simulink model "generating_a_ramp"  (Simulink 6.6)
settings: Solver=VariableStepDiscrete  SolverMode=SingleTasking  StartTime=0.0  StopTime=2048/100e3  RelTol=1e-3
libraries: xbsIndex_r4 x5
settings Model: Creator=lcrockett  LastModifiedBy=lcrockett
settings DataIOCC: SignalLoggingName=sigsOut
settings OptimizationCC: InlineParams=on  InlineInvariantSignals=on
settings DebuggingCC: SignalResolutionControl=TryResolveAllWithWarning  SolverPrmCheckMsg=none  MultiTaskDSMMsg=warning  MultiTaskCondExecSysMsg=none  StrictBusMsg=None
settings HardwareCC: TargetUnknown=on
settings RTWCC: IncludeERTFirstTime=on
settings GRTTargetCC: ModelReferenceCompliant=off  MatFileLogging=off

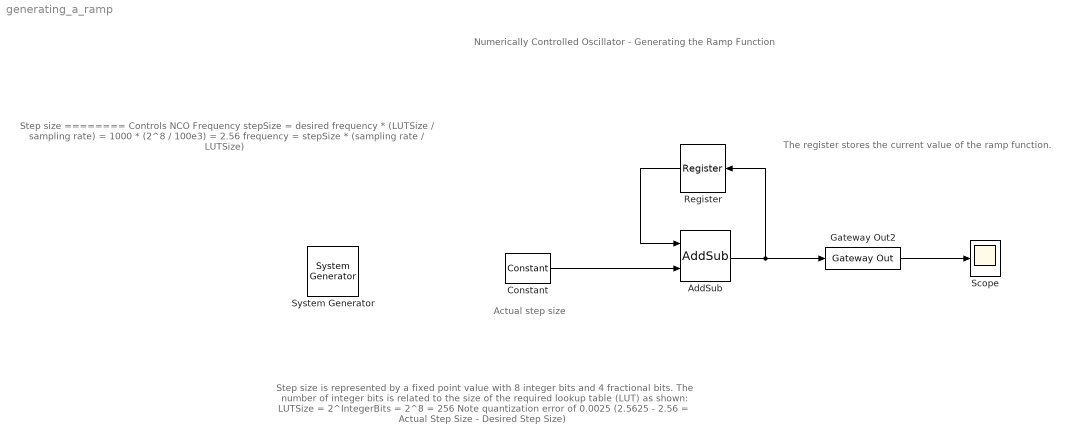
== system generating_a_ramp ==
  note: Step size
      | ========
      | Controls NCO Frequency
      |
      | stepSize =  desired frequency * (LUTSize  / sampling rate)
      |               =  1000 * (2^8  / 100e3)
      |               =  2.56
      |
      | frequency = stepSize * (sampling rate / LUTSize)
  note: The register stores the current value of the ramp function.
  note: Numerically Controlled Oscillator - Generating the Ramp Function
  note: Actual step size
  note: Step size is represented by a fixed point value with 8 integer bits and 4 fractional bits.
      | The number of integer bits is related to the size of the required lookup table (LUT) as shown:
      |
      | LUTSize = 2^IntegerBits = 2^8 = 256
      |
      | Note quantization error of 0.0025 (2.5625 - 2.56 = Actual Step Size - Desired Step Size)
  " System Generator" : xbsIndex_r4/ System Generator  Tag=genX  SystemSampleTime=-1  xilinxfamily=virtex2p  part=xc2vp30  speed=-7  package=ff896  synthesis_tool=XST  directory=./netlist  testbench=off  simulink_period=1/100e3  sysclk_period=50  incr_netlist=off  trim_vbits=Everywhere in SubSystem  dbl_ovrd=According to Block Masks  core_generation=According to Block Masks  run_coregen=off  deprecated_control=off  eval_field=0  block_type=sysgen
      settings: block_version=9.2.01
  AddSub : xbsIndex_r4/AddSub  mode=Addition  use_carryin=off  use_carryout=off  en=off  latency=0  precision=User Defined  arith_type="Signed  (2's comp)"  n_bits=12  bin_pt=4  quantization=Truncate  overflow=Wrap  dbl_ovrd=off  use_behavioral_HDL=on  pipelined=off  use_rpm=on  block_type=addsub
      settings: xl_area=[0, 0, 0, 0, 0, 0, 0]  block_version=VER_STRING_GOES_HERE
  Constant : xbsIndex_r4/Constant  arith_type=Signed (2's comp)  const=2.56  n_bits=12  bin_pt=4  explicit_period=on  period=1/100e3  equ=P=C  opselect=C  inp2=PCIN>>17  opr=+  inp1=P  carry=CIN  dbl_ovrd=off  block_type=constant
      settings: block_version=VER_STRING_GOES_HERE
  Gateway Out2 : xbsIndex_r4/Gateway Out  hdl_port=on  timing_constraint=None  locs_specified=off  LOCs={}  block_type=gatewayout
      settings: infoedit="Gateway out block.  Converts Xilinx fixed point inputs into ouputs of type Simulink integer, double, or fixed point.<P><P>Hardware notes:  In hardware these blocks become top level output ports or are discarded, depending on how they are configured."  xl_area=[0, 0, 0, 0, 0, 0, 0]  block_version=VER_STRING_GOES_HERE
  Register : xbsIndex_r4/Register  Orientation=left  init=0  rst=off  en=off  dbl_ovrd=off  block_type=register
      settings: xl_area=[0, 0, 0, 0, 0, 0, 0]  block_version=VER_STRING_GOES_HERE
  Scope : Scope
      settings: TimeRange=8e-006  YMin=-10000  YMax=10000
  wires:
  Constant/1 -> AddSub/2
  AddSub/1 -> Register/1, Gateway Out2/1
  Register/1 -> AddSub/1
  Gateway Out2/1 -> Scope/1
